simulink model "dft_bank_3"  (Simulink 7.8)
settings: Solver=ode45  StartTime=0.0  StopTime=10.0  RelTol=1e-3
values from neighbouring files (symbols this model uses):
  N = 2    [CFIR_1.m]    (also in TP_fdesign2.m = 128; cic_dezim1.m = ',num2str(N),')']); cic_dezim1_.m = ', num2str(N),' Gain = ',num2str(Hm.gain)]); cic_dezim2.m = ',num2str(N),')']))
  Ts = 1/fs    (= 6.25e-05)    [G722_1.m]    (also in adaptiv_2.m = 0.001; adaptiv_3.m = 0.001; adaptiv_4.m = 0.001; adaptiv_5.m = 0.001)
undefined symbols (not defined in the file or in its folder): Ksub, WN, WNt
libraries: dspsigops x1, dspobslib x1, simulink x1
settings Model: Creator=svenhoffmann  LastModifiedBy=josef  ExtModeAutoUpdateStatusClock=off
settings DataIOCC: SignalLoggingName=sigsOut
settings OptimizationCC: InitFltsAndDblsToZero=on
settings DebuggingCC: SaveWithParameterizedLinksMsg=none  SignalResolutionControl=TryResolveAllWithWarning  SolverPrmCheckMsg=none  MultiTaskDSMMsg=warning  MultiTaskCondExecSysMsg=none  FcnCallInpInsideContextMsg=Use local settings  StrictBusMsg=None
settings HardwareCC: TargetUnknown=on
settings RTWCC: IncludeERTFirstTime=on
settings GRTTargetCC: TargetFcnLib=ansi_tfl_tmw.mat

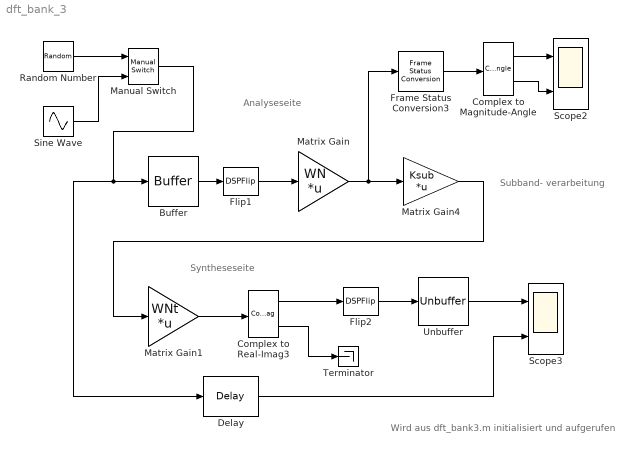
== system dft_bank_3 ==
  note: Analyseseite
  note: Syntheseseite
  note: Subband-
      | verarbeitung
  note: Wird aus dft_bank3.m initialisiert und aufgerufen
  Buffer : Buffer  N=N
  Complex to Magnitude-Angle : ComplexToMagnitudeAngle
  Complex to Real-Imag3 : ComplexToRealImag
  Delay : dspsigops/Delay  InputProcessing=Inherited (this choice will be removed - see release notes)  dly_unit=Samples  delay=10  ic_detail=off  dif_ic_for_ch=off  dif_ic_for_dly=off  ic=0  reset_popup=None
  Flip1 : DSPFlip
  Flip2 : DSPFlip
  Frame Status Conversion3 : dspobslib/Frame Status Conversion  growRefPort=off  outframe=Sample-based
  Manual Switch : simulink/Signal Routing/Manual Switch  sw=1  action=0  varsize=off
  Matrix Gain : Gain  Gain=WN  Multiplication=Matrix(K*u)  SaturateOnIntegerOverflow=on  OutDataTypeStr=Inherit: Same as input  ParamDataTypeStr=Inherit: Same as input
  Matrix Gain1 : Gain  Gain=WNt  Multiplication=Matrix(K*u)  SaturateOnIntegerOverflow=on  OutDataTypeStr=Inherit: Same as input  ParamDataTypeStr=Inherit: Same as input
  Matrix Gain4 : Gain  Gain=Ksub  Multiplication=Matrix(K*u)  SaturateOnIntegerOverflow=on  OutDataTypeStr=Inherit: Same as input  ParamDataTypeStr=Inherit: Same as input
  Random Number : RandomNumber  SampleTime=Ts
  Scope2 : Scope  NumInputPorts=2
      settings: TimeRange=0.2  YMin=-8.32667e-17~-3  YMax=0.65~3.5
  Scope3 : Scope  NumInputPorts=2
      settings: TimeRange=1  YMin=-1~-1  YMax=1~1
  Sine Wave : Sin  Frequency=2*pi*100  SampleTime=Ts
  Terminator : Terminator
  Unbuffer : Unbuffer
  wires:
  Buffer/1 -> Flip1/1
  Flip1/1 -> Matrix Gain/1
  Matrix Gain/1 -> Frame Status Conversion3/1, Matrix Gain4/1
  Matrix Gain1/1 -> Complex to Real-Imag3/1
  Complex to Real-Imag3/1 -> Flip2/1
  Complex to Real-Imag3/2 -> Terminator/1
  Delay/1 -> Scope3/2
  Matrix Gain4/1 -> Matrix Gain1/1
  Complex to Magnitude-Angle/1 -> Scope2/1
  Complex to Magnitude-Angle/2 -> Scope2/2
  Frame Status Conversion3/1 -> Complex to Magnitude-Angle/1
  Flip2/1 -> Unbuffer/1
  Unbuffer/1 -> Scope3/1
  Random Number/1 -> Manual Switch/1
  Sine Wave/1 -> Manual Switch/2
  Manual Switch/1 -> Buffer/1, Delay/1
